simulink subsystem "Guide_Flight_Path_Energy"  (R2025b)
settings: Solver=VariableStepAuto  StartTime=0.0  StopTime=10.0  RelTol=1e-3
settings Model: Creator=invrt  LastModifiedBy=invrt

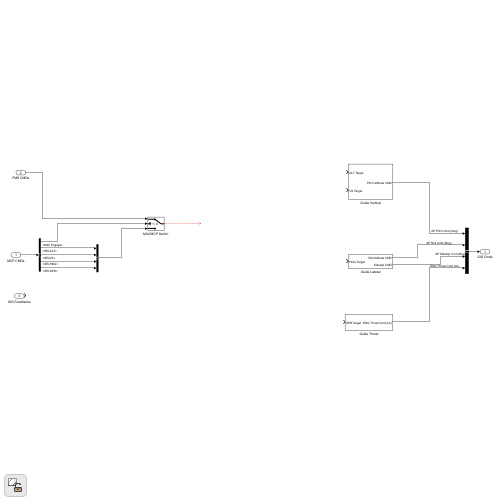
[thumbnail: Simulink's stored preview of the top-level diagram]
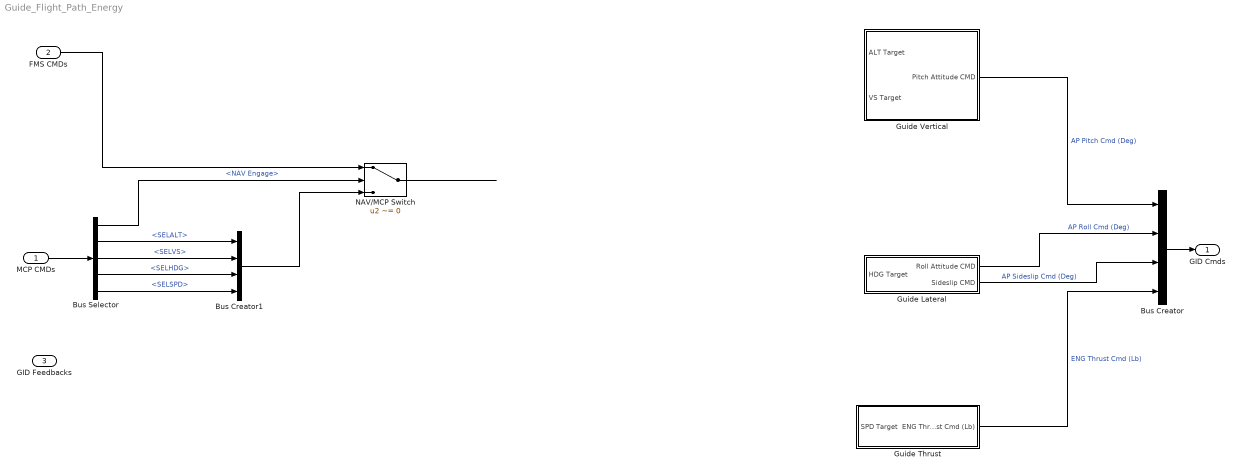
== system Guide_Flight_Path_Energy ==
  MCP CMDs : Inport
  FMS CMDs : Inport  Port=2
  GID Feedbacks : Inport  Port=3
  Bus Creator : BusCreator  Inputs=4
  Bus Creator1 : BusCreator  Inputs=4
  Bus Selector : BusSelector  OutputSignals=NAV Engage,Vert GID Bus.SELALT,Vert GID Bus.SELVS,Lat GID Bus.SELHDG,Spd/Mach GID Bus.SELSPD
  Guide Lateral : Subsystem
  Guide Thrust : Subsystem
  Guide Vertical : Subsystem
  NAV/MCP Switch : Switch  Criteria=u2 ~= 0  SaturateOnIntegerOverflow=off  InputSameDT=off
  GID Cmds : Outport
  wires:
  Guide Vertical/1(Pitch Attitude CMD) -> Bus Creator/1  "AP Pitch Cmd (Deg)"
  Guide Lateral/1(Roll Attitude CMD) -> Bus Creator/2  "AP Roll Cmd (Deg)"
  Guide Lateral/2(Sideslip CMD) -> Bus Creator/3  "AP Sideslip Cmd (Deg)"
  Guide Thrust/1(ENG Thrust Cmd (Lb)) -> Bus Creator/4  "ENG Thrust Cmd (Lb)"
  Bus Creator/1 -> GID Cmds/1
  MCP CMDs/1 -> Bus Selector/1
  Bus Selector/1 -> NAV/MCP Switch/2  "<NAV Engage>"
  Bus Selector/2 -> Bus Creator1/1  "<SELALT>"
  Bus Selector/3 -> Bus Creator1/2  "<SELVS>"
  Bus Selector/4 -> Bus Creator1/3  "<SELHDG>"
  Bus Selector/5 -> Bus Creator1/4  "<SELSPD>"
  FMS CMDs/1 -> NAV/MCP Switch/1
  Bus Creator1/1 -> NAV/MCP Switch/3
  NAV/MCP Switch/1 -> ?

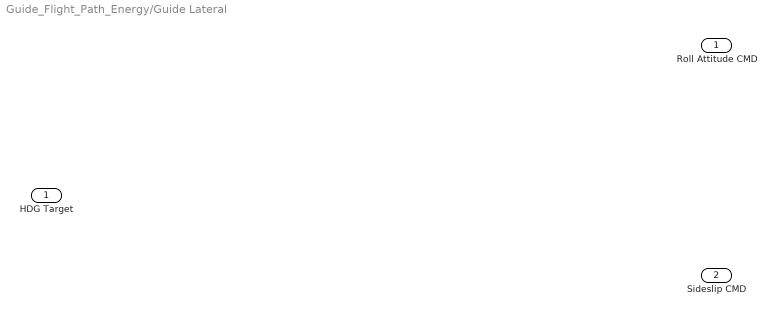
== system Guide_Flight_Path_Energy/Guide Lateral ==
  HDG Target : Inport
  Roll Attitude CMD : Outport
  Sideslip CMD : Outport  Port=2

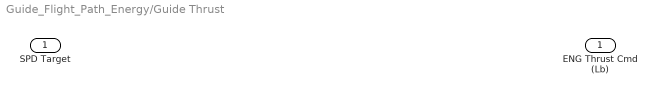
== system Guide_Flight_Path_Energy/Guide Thrust ==
  SPD Target : Inport
  ENG Thrust Cmd (Lb) : Outport

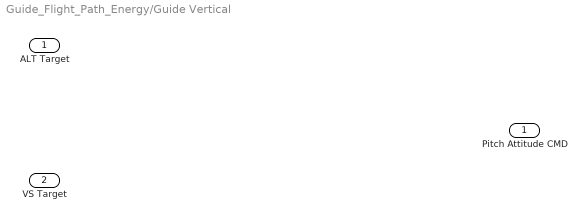
== system Guide_Flight_Path_Energy/Guide Vertical ==
  ALT Target : Inport
  VS Target : Inport  Port=2
  Pitch Attitude CMD : Outport
